simulink model "rtwdemo_counter"  (Simulink 6.0)
settings: Solver=FixedStepDiscrete  StartTime=0.0  StopTime=48  FixedStep=1  RelTol=1e-3
PostLoadFcn:
  | INC=uint8(1);LIMIT=uint8(16);RESET=uint8(0);K=int32(2);
libraries: rtwdemowidgets x2
settings Model: CovMetricSettings=d  Creator=The MathWorks Inc.  LastModifiedBy=batserve  ParamWorkspaceSource=ReferencedWorkspace  ExtModeTrigMode=oneshot  ExtModeArmWhenConnect=off  ExtModeAutoUpdateStatusClock=off
settings DataIOCC: LimitDataPoints=off  SaveFormat=StructureWithTime  SaveOutput=off  SaveTime=off  SignalLoggingName=sigsOut
settings OptimizationCC: InlineParams=on  EnforceIntegerDowncast=off  StateBitsets=on  DataBitsets=on  UseTempVars=on
settings DebuggingCC: CheckExecutionContextPreStartOutputMsg=on  CheckExecutionContextRuntimeOutputMsg=on  SolverPrmCheckMsg=none  IntegerOverflowMsg=none
settings ModelReferenceCC: UpdateModelReferenceTargets=IfOutOfDate
settings RTWCC: TLCOptions=-p0 -aWarnNonSaturatedBlocks=0  GenerateReport=on  RTWVerbose=off  ProcessScript=grt_make_rtw_hook  LaunchReport=on
settings CodeAppCC: ForceParamTrailComments=on  PrefixModelToSubsysFcnNames=off
settings GRTTargetCC: MatFileLogging=off

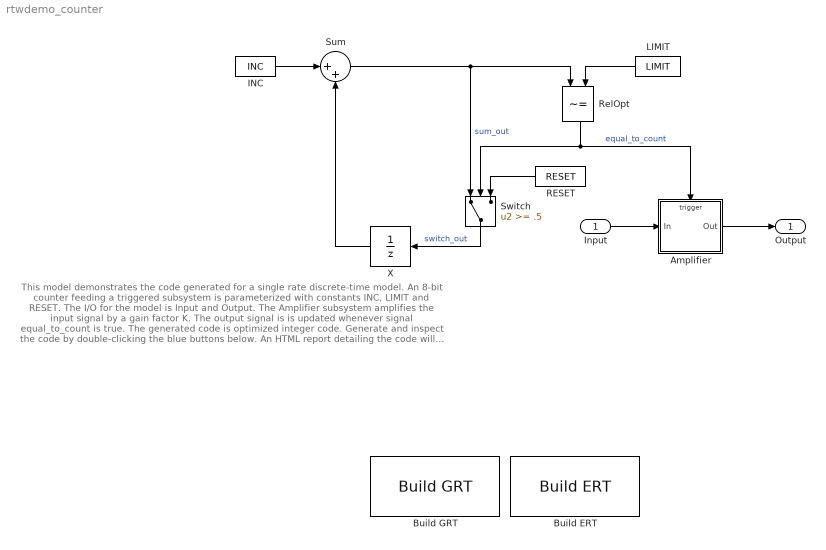
== system rtwdemo_counter ==
  note: This model demonstrates the code generated for a single rate discrete-time model.  An 8-bit
      | counter feeding a triggered subsystem is parameterized with constants INC, LIMIT and RESET.
      | The I/O for the model is Input and Output. The Amplifier subsystem amplifies the input signal
      | by a gain factor K. The output signal is is updated whenever signal equal_to_count  is true.
      | The generated code is optimized integer code.
      |
      | Generate and inspect the code by double-clicking the blue buttons below.  An HTML report
      | detailing the code will be displayed automatically.
  Input : Inport  Port=1  DataType=int32  LatchInput=off
  Amplifier : Subsystem  TreatAsAtomicUnit=on  PropExecContextAcrossSSBoundary=on
  Build ERT : rtwdemowidgets/Build ERT  attrib_overrides={}
  Build GRT : rtwdemowidgets/Build GRT  attrib_overrides={}
  INC : Constant  Value=INC
  LIMIT : Constant  Orientation=left  Value=LIMIT
  RESET : Constant  Orientation=left  Value=RESET
  RelOpt : RelationalOperator  Orientation=down  Operator=~=  InputSameDT=on
  Sum : Sum  Inputs=|++  InputSameDT=on
  Switch : Switch  Orientation=down  Threshold=.5  SaturateOnIntegerOverflow=on  InputSameDT=on
  X : UnitDelay  Orientation=left  StateIdentifier=X
  Output : Outport
  wires:
  INC/1 -> Sum/1
  X/1 -> Sum/2
  Switch/1 -> X/1  "switch_out"
  Sum/1 -> Switch/1, RelOpt/1  "sum_out"
  LIMIT/1 -> RelOpt/2
  Input/1 -> Amplifier/1(In)
  RESET/1 -> Switch/3
  RelOpt/1 -> Switch/2, Amplifier/Trigger  "equal_to_count"
  Amplifier/1(Out) -> Output/1

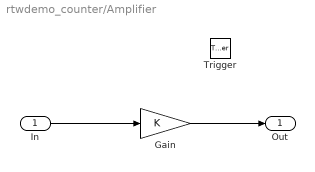
== system rtwdemo_counter/Amplifier ==
  In : Inport  Port=1  LatchInput=off
  Trigger : TriggerPort
  Gain : Gain  Gain=K
  Out : Outport  InitialOutput=0
  wires:
  In/1 -> Gain/1
  Gain/1 -> Out/1
